simulink model "Phase1_Mark2"  (R2024b)
settings: Solver=ode23tb  StartTime=0.0  StopTime=inf  FixedStep=.001  RelTol=1e-1
model workspace (MAT data in the model file):
  A_mu = 10
  B_reff = 8.386
  CONVERTER_DATA = [0 0.1 0.2 0.3 0.4 0.5 0.6 0.7 0.8 0.81 0.82 0.83 ... (63 elements, 21x3)]
  Cps = 2
  Cz = 7766.25
  DOWN_TABLE = [0 0 0 0 0 0 5 5 7.5 7.5 15 15 ... (30 elements, 6x5)]
  DOWN_TH_BP = [0 5 40 50 90 100]
  D_reff = 0.25826
  EMAP = [-40 215 245 264 264 267 267 267 267 267 -44 117 ... (110 elements, 10x11)]
  F0z = [6086.4 4324.8]
  F_reff = 0.07394
  F_zmax = 10000
  F_zmin = 100
  F_zo = 4000
  Kz = 48000
  MF : object (value not decoded)
  NCyl = 6
  NE_VEC = [800 1200 1600 2000 2400 2800 3200 3600 4000 4400 4800]
  Pstd = 101325
  Rair = 287
  SUS : object (value not decoded)
  TH_VEC = [0; 20; 30; 40; 50; 60; 70; 80; 90; 100]
  TWAITdn = 1.25
  TWAITup = 0.1
  Tin = [1 2 3 4 5 6 7 8 9 10 2 2 ... (20 elements, 10x2)]
  Tstd = 293.15
  UP_TABLE = [7.5 7.5 15 25 40 40 25 25 35 45 70 80 ... (30 elements, 6x5)]
  UP_TH_BP = [0 25 35 50 90 100]
  VEH : object (value not decoded)
  V_o = 16.7
  V_xlow = 1
  Vd = 0.00346
  WH : object (value not decoded)
  a = 1.515
  alpha_max = 1.5
  alpha_min = -1.5
  b = 1.504
  c_zo = 209651
  epsilon = 0.1
  f_air = [0 0 0 0 0 0 0 0 0 0 0 0 ... (256 elements, 16x16)]
  f_co = [0 0 0 0 0 0 0 0 0 0 0 0 ... (256 elements, 16x16)]
  f_co2 = [0 0 0 0 0 0 0 0 0 0 0 0 ... (256 elements, 16x16)]
  f_eff = [352.135682859 352.135682859 320.724378192 303.655312657 295.930136708 291.240087194 291.240271258 291.240312459 291.240275452 291.240198499 291.240100781 291.240018769 ... (256 elements, 16x16)]
  f_fuel = [0 0 0 0 0 0 0 0 0 0 0 0 ... (256 elements, 16x16)]
  f_hc = [0 0 0 0 0 0 0 0 0 0 0 0 ... (256 elements, 16x16)]
  f_nox = [0 0 0 0 0 0 0 0 0 0 0 0 ... (256 elements, 16x16)]
  f_pm = [0 0 0 0 0 0 0 0 0 0 0 0 ... (256 elements, 16x16)]
  f_susp_axl_bp = [1 2]
  f_susp_dz_bp = [-4 -0.14 -0.13 -0.12 -0.11 -0.1 -0.09 -0.08 -0.07 -0.06 -0.05 -0.04 ... (31 elements, 1x31)]
  f_susp_dzdot_bp = [-4 -0.14 -0.13 -0.12 -0.11 -0.1 -0.09 -0.08 -0.07 -0.06 -0.05 -0.04 ... (31 elements, 1x31)]
  f_susp_fmz = [-213379.591456 -28099.591456 -27619.591456 -27139.591456 -26659.591456 -26179.591456 -25699.591456 -25219.591456 -24739.591456 -24259.591456 -23779.591456 -23299.591456 ... (468968 elements, 31x31x61x2x4)]
  f_susp_geom = [-0.832564012244 0.043269987756 0.045538987756 0.047807987756 0.050076987756 0.052345987756 0.054614987756 0.056883987756 0.059152987756 0.061421987756 0.063690987756 0.065959987756 ... (11346 elements, 31x61x2x3)]
  f_susp_strgdelta_bp = [-0.523598775598 -0.506145483078 -0.488692190558 -0.471238898038 -0.453785605519 -0.436332312999 -0.418879020479 -0.401425727959 -0.383972435439 -0.366519142919 -0.349065850399 -0.331612557879 ... (61 elements, 1x61)]
  f_tbrake = [0 76.8593923996 105.140482948 131.533638111 157.926793274 176.658631717 176.65727296 176.656856686 176.656879077 176.657093756 176.657404516 176.65772406 ... (256 elements, 16x16)]
  f_tbrake_n_bpt = [0 649.519052838 912.419621844 1175.32019085 1438.22075986 1701.12132886 1964.02189787 2226.92246687 2489.82303588 2752.72360489 3015.62417389 3278.5247429 ... (16 elements, 1x16)]
  f_tbrake_t_bpt = [0 34.6410161514 61.0341713143 87.4273264773 113.82048164 140.213636803 166.606791966 192.999947129 219.393102292 245.786257455 272.179412618 298.572567781 ... (16 elements, 1x16)]
  f_texh = [766.752464599 766.752464599 786.17542386 801.679939032 884.591982581 910.574397722 910.571871054 910.570774534 910.570601632 910.570821151 910.571247242 910.571639815 ... (256 elements, 16x16)]
  f_twc_eff_co = [0.17 0.25 0.45 0.99 0.99 0.99 0.99]
  f_twc_eff_hc = [0.21 0.375 0.75 0.98 0.98 0.98 0.98]
  f_twc_eff_lam = [0.909090909 0.944055944 0.979020979 1 1.013986014 1.048951049 1.083916084]
  f_twc_eff_nox = [0.98 0.98 0.98 0.97 0.05 0.02 0]
  h = 0.134
  k_z = 50
  kappa_max = 1.5
  kappa_min = -1.5
  lam_Cx = 1
  lam_Cy = 1
  lam_Cz = 1
  lam_Ex = 1
  lam_Ey = 1
  lam_F_zo = 1
  lam_Hx = 1
  lam_Hy = 1
  lam_Kxkappa = 1
  lam_Kyalpha = 1
  lam_Kygamma = 1
  lam_Kzgamma = 1
  lam_Mr = 1
  lam_Mx = 1
  lam_My = 1
  lam_S = 1
  lam_VMx = 1
  lam_Vx = 1
  lam_Vy = 1
  lam_Vykappa = 1
  lam_muV = 0
  lam_mux = 1
  lam_muy = 1
  lam_t = 1
  lam_xalpha = 1
  lam_ykappa = 1
  numWheel = 4
  p_Cx1 = 1.579
  p_Cy1 = 1.3332
  p_Dx1 = 1.0422
  p_Dx2 = -0.08285
  p_Dx3 = 0
  p_Dy1 = 0.8784
  p_Dy2 = -0.06445
  p_Dy3 = 0
  p_Ex1 = 0.11185
  p_Ex2 = 0.3127
  p_Ex3 = 0
  p_Ex4 = 0.001603
  p_Ey1 = -0.8227
  p_Ey2 = -0.6062
  p_Ey3 = 0.09825
  p_Ey4 = -6.546
  p_Ey5 = 0
  p_Fz1 = 0.7098
  p_Hx1 = 0.00021585
  p_Hx2 = 0.0011538
  p_Hy1 = -0.0018043
  p_Hy2 = 0.003518
  p_Kx1 = 21.69
  p_Kx2 = 13.774
  p_Kx3 = -0.4119
  p_Ky1 = -15.314
  p_Ky2 = 1.7044
  p_Ky3 = 0.36986
  p_Ky4 = 1.9896
  p_Ky5 = 0
  p_Ky6 = -0.9004
  p_Ky7 = -0.2328
  p_Vx1 = 1.5973e-05
  p_Vx2 = 0.0001043
  p_Vy1 = -0.006642
  p_Vy2 = 0.03597
  p_Vy3 = -0.1621
  p_Vy4 = -0.4908
  p_pmx1 = 0
  p_px1 = -0.3489
  p_px2 = 0.382
  p_px3 = -0.09634
  p_px4 = 0.06447
  p_py1 = -0.6249
  p_py2 = -0.06535
  p_py3 = -0.1668
  p_py4 = 0.2834
  p_py5 = 0
  path : object (value not decoded)
  pio = 220000
  q_Fcx = 0
  q_Fz2 = 15.4
  q_Fzy = 0
  q_reo = 0.9974
  q_sx1 = -0.007764
  q_sx10 = 0.2824
  q_sx11 = 5.349
  q_sx12 = 0
  q_sx13 = 0
  q_sx14 = 0
  q_sx2 = 1.1915
  q_sx3 = 0.013948
  q_sx4 = 4.912
  q_sx5 = 1.02
  q_sx6 = 22.83
  q_sx7 = 0.7104
  q_sx8 = -0.023393
  q_sx9 = 0.6581
  q_sy1 = 0.00702
  q_sy2 = 0
  q_sy3 = 0.001515
  q_sy4 = 8.514e-05
  q_sy5 = 0
  q_sy6 = 0
  q_sy7 = 0.9008
  q_sy8 = -0.4089
  q_v1 = 0.0007742
  q_v2 = 0.04667
  r_Bx1 = 12.531
  r_Bx2 = 9.532
  r_Bx3 = 0
  r_By1 = 10.615
  r_By2 = 7.705
  r_By3 = 3.433e-06
  r_By4 = 0
  r_Cx1 = 1.019
  r_Cy1 = 1.0585
  r_Ex1 = -0.4487
  r_Ex2 = -0.4726
  r_Ey1 = 0.3132
  r_Ey2 = 7.63e-06
  r_Hx1 = 0.0002374
  r_Hy1 = 0.011646
  r_Hy2 = 7.63e-06
  r_Vy1 = 0.05654
  r_Vy2 = 7.63e-06
  r_Vy3 = 0
  r_Vy4 = 99.9
  r_Vy5 = 2
  r_Vy6 = 15.814
  r_o = 0.3135
  reqTmaxT = [nan 0.285774810084 0.647179872268 nan nan nan nan nan nan nan nan nan ... (168 elements, 21x8)]
  vehSpd = [0 2.77777777778 5.55555555556 8.33333333333 11.1111111111 13.8888888889 16.6666666667 19.4444444444 22.2222222222 25 27.7777777778 30.5555555556 ... (21 elements, 1x21)]
  vehWidth = 2
  w = 1
symbols that are objects in the model workspace (value not decoded): VEH
undefined symbols (not defined in the file or in its folder): Fzz, Fzzdot, InertFrm, pFz, psi, vdyntiremask, x_o, zdotFz, zFz
(part 13 of 24)

== system Phase1_Mark2/Vehicle Body 3DOF External Longitudinal Wheels/Dual/Vehicle Body 3DOF Dual Track/Signal Routing/Signal Routing Dual/state2bus ==
  x : Inport
  y : Inport  Port=2
  Xo : Inport  Port=3
  Angle Wrap : Subsystem  Variant=on  VariantControlMode=label  VariantControl=Variant1  LabelModeActiveChoice=Wrap
  Body Slip : Subsystem
  Bus Creator1 : BusCreator  Inputs=6
  Bus Creator{3,6..7,10..11,13..14} (7 alike) : BusCreator  Inputs=3
  Bus Creator15 : BusCreator  Inputs=6
  Bus Creator2 : BusCreator  Inputs=1
  COMB2I : MATLAB Function  TreatAsAtomicUnit=on
  Constant{,1..10} (11 alike) : Constant  Value=0
  Demux{1..2,4,6} (4 alike) : Demux  Outputs=2
  Demux3 : Demux  Outputs=3
  Demux5 : Demux  Outputs=3
  Integrator : Integrator  InitialConditionSource=external
  Rotation Angles to Direction Cosine Matrix : Subsystem  mask(Ang2DCM){rotationOrder=ZYX, aMode=aMode}
      mask prompts: rotationOrder "shared_aeroblks:sharedaeroblktransform:blockAng2DCMParamRotationOrder"
      mask help: shared_aeroblks:sharedaeroblktransform:blockAng2DCMDesc
      mask init:
      | if aerosharedtest(gcb)
      |     ports=aerosharedicon('sharedang2dcm');
      | else
      |     ports=sharedautoicon('sharedang2dcm');
      | end
      settings: AttributesFormatString=Rotation Order: %<rotationOrder>
      mask Help: eval('if license(''test'',''Aerospace_Blockset'')aerosharedhelp(''rotation_angles_to_direction_cosine_matrix'');elseif license(''test'',''Powertrain_Blockset'')sharedautohelp(''rotation_angles_to_direction_cosine_matrix'');end')
      mask TypeOptions rotationOrder: shared_aeroblks:sharedaeroblktransform:blockParamComboZYX | shared_aeroblks:sharedaeroblktransform:blockParamComboZYZ | shared_aeroblks:sharedaeroblktransform:blockParamComboZXY | shared_aeroblks:sharedaeroblktransform:blockParamComboZXZ | shared_aeroblks:sharedaeroblktransform:blockParamComboYXZ | shared_aeroblks:sharedaeroblktransform:blockParamComboYXY | shared_aeroblks:sharedaeroblktransform:blockParamComboYZX | shared_aeroblks:sharedaeroblktransform:blockParamComboYZY | shared_aeroblks:sharedaeroblktransform:blockParamComboXYZ | shared_aeroblks:sharedaeroblktransform:blockParamComboXYX | shared_aeroblks:sharedaeroblktransform:blockParamComboXZY | shared_aeroblks:sharedaeroblktransform:blockParamComboXZX
      mask DialogControl rotationOrder Prompt: Rotation order:
      mask Display:
      | port_label('input',1,'[R_1,R_2,R_3]','texmode','on')
      | port_label('output',1,'DCM_{be}','texmode','on')
  Selector : Selector  InputPortWidth=3  IndexOptions=Index vector (dialog)  Indices=[3 2 1]  OutputSizes=1
  Selector1 : Selector  IndexOptions=Index vector (dialog)  Indices=[3]  OutputSizes=1
  Selector2 : Selector  IndexOptions=Index vector (dialog)  Indices=[3,1,2]  OutputSizes=1
  Selector4 : Selector  IndexOptions=Index vector (dialog)  Indices=[4,1,2]  OutputSizes=1
  Selector5 : Selector  IndexOptions=Index vector (dialog)  Indices=[1,2]  OutputSizes=1
  Signal Specification : SignalSpecification  Unit=gn
  Signal Specification1 : SignalSpecification  Unit=rad/s
  Signal Specification{4..6,10..12} (6 alike) : SignalSpecification  Unit=m/s
  Signal Specification13 : SignalSpecification  Unit=m
  Signal Specification14 : SignalSpecification  Unit=m
  Signal Specification15 : SignalSpecification  Unit=m
  Signal Specification16 : SignalSpecification  Unit=m/s^2
  Signal Specification17 : SignalSpecification  Unit=m/s^2
  Signal Specification18 : SignalSpecification  Unit=m/s^2
  Signal Specification19 : SignalSpecification  Unit=rad/s^2
  Signal Specification2 : SignalSpecification  Unit=rad/s
  Signal Specification20 : SignalSpecification  Unit=rad/s^2
  Signal Specification21 : SignalSpecification  Unit=rad/s^2
  Signal Specification3 : SignalSpecification  Unit=rad/s
  Signal Specification7 : SignalSpecification  Unit=rad
  Signal Specification8 : SignalSpecification  Unit=rad
  Signal Specification9 : SignalSpecification  Unit=rad
  xddot2ax : Subsystem
  COM_I : Outport  VectorParamsAs1DForOutWhenUnconnected=off
  COM_B : Outport  Port=2  VectorParamsAs1DForOutWhenUnconnected=off
  wires:
  Rotation Angles to Direction Cosine Matrix/1(Out1) -> Bus Creator15/6  "DCM"
  Selector/1 -> Rotation Angles to Direction Cosine Matrix/1(In1)
  [angles] -> Selector/1
  Angle Wrap/1(" y") -> Signal Specification7/1
  Constant10/1 -> Signal Specification20/1
  Bus Creator3/1 -> Bus Creator15/5  "AngAcc"
  Constant9/1 -> Signal Specification19/1
  Signal Specification20/1 -> Bus Creator3/1  "pdot"
  Selector1/1 -> Signal Specification21/1
  Signal Specification19/1 -> Bus Creator3/2  "qdot"
  Signal Specification21/1 -> Bus Creator3/3  "rdot"
  Xo/1 -> Integrator/2
  Bus Creator2/1 -> Bus Creator15/2  "Ang"
  Body Slip/1(Beta) -> Bus Creator2/1  "Beta"
  Demux6/2 -> Signal Specification17/1
  Demux6/1 -> Signal Specification16/1
  Signal Specification16/1 -> Bus Creator1/4  "xddot"
  Signal Specification18/1 -> Bus Creator1/6  "zddot"
  Signal Specification17/1 -> Bus Creator1/5  "yddot"
  Bus Creator1/1 -> Bus Creator15/4  "Acc"
  xddot2ax/1(ax) -> Bus Creator1/1  "ax"
  Demux5/1 -> xddot2ax/1(r), Signal Specification1/1  "r"
  xddot2ax/2(ay) -> Bus Creator1/2  "ay"
  Selector5/1 -> Demux6/1, Demux4/1
  Demux4/2 -> xddot2ax/5(yddot)  "yddot"
  Constant3/1 -> Signal Specification18/1  "zddot"
  Signal Specification/1 -> Bus Creator1/3  "az"
  Demux5/3 -> xddot2ax/3(ydot)  "ydot"
  Constant1/1 -> Signal Specification/1  "az"
  Selector4/1 -> Demux5/1
  Demux4/1 -> xddot2ax/4(xddot)  "xddot"
  Demux5/2 -> xddot2ax/2(xdot)  "xdot"
  y/1 -> Selector5/1, Selector1/1
  Demux2/1 -> Signal Specification14/1
  Demux2/2 -> Signal Specification15/1
  Constant/1 -> Signal Specification13/1
  Demux1/1 -> Signal Specification11/1
  Demux1/2 -> Signal Specification12/1
  Constant8/1 -> Signal Specification10/1
  Constant2/1 -> Signal Specification9/1
  Constant7/1 -> Signal Specification8/1
  Demux3/1 -> Angle Wrap/1("u ")
  Demux3/3 -> Signal Specification6/1
  Demux3/2 -> Signal Specification5/1
  Constant6/1 -> Signal Specification4/1
  Constant4/1 -> Signal Specification3/1
  Constant5/1 -> Signal Specification2/1
  Signal Specification1/1 -> Bus Creator13/3  "r"
  x/1 -> Selector4/1, Body Slip/1(x), Selector2/1, COMB2I/1(x)
  Signal Specification10/1 -> Bus Creator6/3  "Zdot"
  Signal Specification4/1 -> Bus Creator14/3  "zdot"
  Signal Specification11/1 -> Bus Creator6/1  "Xdot"
  Signal Specification15/1 -> Bus Creator10/2  "Y"
  Bus Creator13/1 -> Bus Creator15/3  "AngVel"
  Signal Specification13/1 -> Bus Creator10/3  "Z"
  Signal Specification14/1 -> Bus Creator10/1  "X"
  Signal Specification9/1 -> Bus Creator11/1  "phi"
  Bus Creator7/1 -> COM_I/1  "COM_I"
  Signal Specification3/1 -> Bus Creator13/1  "p"
  Bus Creator14/1 -> Bus Creator15/1  "Vel"
  Bus Creator6/1 -> Bus Creator7/2  "Vel"
  Bus Creator10/1 -> Bus Creator7/1  "Disp"
  Signal Specification8/1 -> Bus Creator11/2  "theta"
  Selector2/1 -> Demux3/1
  Signal Specification12/1 -> Bus Creator6/2  "Ydot"
  Signal Specification2/1 -> Bus Creator13/2  "q"
  Bus Creator15/1 -> COM_B/1  "COM_B"
  Signal Specification5/1 -> Bus Creator14/1  "xdot"
  Bus Creator11/1 -> Bus Creator7/3, [angles]  "Ang"
  Signal Specification6/1 -> Bus Creator14/2  "ydot"
  Integrator/1 -> Demux2/1
  COMB2I/1(y) -> Integrator/1, Demux1/1
  Signal Specification7/1 -> Bus Creator11/3  "psi"

== system Phase1_Mark2/Vehicle Body 3DOF External Longitudinal Wheels/Dual/Vehicle Body 3DOF Dual Track/sigma/sigma/relaxation front ==
  alpha : Inport
  V : Inport  Port=2
  sigma : Inport  Port=3
  Product1 : Product  Inputs=**/  InputSameDT=on  RndMeth=Zero  SaturateOnIntegerOverflow=on  OutDataTypeStr=Inherit: Same as first input
  Sum : Sum  Inputs=-+|  InputSameDT=on  SaturateOnIntegerOverflow=on  OutDataTypeStr=Inherit: Same as first input
  lateral : Integrator
  alpha_sig : Outport  VectorParamsAs1DForOutWhenUnconnected=off
  wires:
  lateral/1 -> alpha_sig/1, Sum/1
  sigma/1 -> Product1/3
  Sum/1 -> Product1/1
  Product1/1 -> lateral/1
  V/1 -> Product1/2
  alpha/1 -> Sum/2

== system Phase1_Mark2/Vehicle Body 3DOF External Longitudinal Wheels/Dual/Vehicle Body 3DOF Dual Track/sigma/sigma/relaxation rear ==
  alpha : Inport
  V : Inport  Port=2
  sigma : Inport  Port=3
  Product1 : Product  Inputs=**/  InputSameDT=on  RndMeth=Zero  SaturateOnIntegerOverflow=on  OutDataTypeStr=Inherit: Same as first input
  Sum : Sum  Inputs=-+|  InputSameDT=on  SaturateOnIntegerOverflow=on  OutDataTypeStr=Inherit: Same as first input
  lateral : Integrator
  alpha_sig : Outport  VectorParamsAs1DForOutWhenUnconnected=off
  wires:
  alpha/1 -> Sum/2
  V/1 -> Product1/2
  Product1/1 -> lateral/1
  Sum/1 -> Product1/1
  sigma/1 -> Product1/3
  lateral/1 -> alpha_sig/1, Sum/1

== system Phase1_Mark2/Vehicle Body 3DOF External Longitudinal Wheels/Dual/Vehicle Body 3DOF Dual Track/sigma/sigma dual/relaxation ==
  alpha : Inport
  V : Inport  Port=2
  sigma : Inport  Port=3
  Product1 : Product  Inputs=**/  InputSameDT=on  RndMeth=Zero  SaturateOnIntegerOverflow=on  OutDataTypeStr=Inherit: Same as first input
  Sum : Sum  Inputs=-+|  InputSameDT=on  SaturateOnIntegerOverflow=on  OutDataTypeStr=Inherit: Same as first input
  lateral : Integrator
  alpha_sig : Outport  VectorParamsAs1DForOutWhenUnconnected=off
  wires:
  alpha/1 -> Sum/2
  V/1 -> Product1/2
  Product1/1 -> lateral/1
  Sum/1 -> Product1/1
  sigma/1 -> Product1/3
  lateral/1 -> Sum/1, alpha_sig/1

== system Phase1_Mark2/Longitudinal Wheels 4DOF/Tires/Fiala/Fiala Tire/Fiala/Rolling/ISO ==
  "Omega " : Inport
  Fz : Inport  Port=2
  Re : Inport  Port=3
  Tamb : Inport  Port=4
  MATLAB Function : MATLAB Function  TreatAsAtomicUnit=on
  My : Outport  VectorParamsAs1DForOutWhenUnconnected=off
  wires:
  Fz/1 -> MATLAB Function/1(Fz)
  "Omega "/1 -> MATLAB Function/2(omega)
  Tamb/1 -> MATLAB Function/3(Tamb)
  Re/1 -> MATLAB Function/4(Re)
  MATLAB Function/1(My) -> My/1

== system Phase1_Mark2/Longitudinal Wheels 4DOF/Tires/Fiala/Fiala Tire/Fiala/Rolling/MagicFormula ==
  "Omega " : Inport
  Fz : Inport  Port=2
  Vx : Inport  Port=3
  Fx : Inport  Port=4
  gamma : Inport  Port=5
  Prs : Inport  Port=6
  MATLAB Function : MATLAB Function  TreatAsAtomicUnit=on
  My : Outport  VectorParamsAs1DForOutWhenUnconnected=off
  wires:
  "Omega "/1 -> MATLAB Function/1(Omega)
  Fz/1 -> MATLAB Function/3(Fz)
  Fx/1 -> MATLAB Function/2(Fx)
  Vx/1 -> MATLAB Function/4(Vx)
  Prs/1 -> MATLAB Function/5(press)
  gamma/1 -> MATLAB Function/6(gamma)
  MATLAB Function/1(My) -> My/1

== system Phase1_Mark2/Longitudinal Wheels 4DOF/Tires/Fiala/Fiala Tire/Fiala/Rolling/Mapped ==
  "Omega " : Inport
  Fz : Inport  Port=2
  Vx : Inport  Port=3
  MATLAB Function : MATLAB Function  TreatAsAtomicUnit=on
  My : Outport  VectorParamsAs1DForOutWhenUnconnected=off
  wires:
  "Omega "/1 -> MATLAB Function/1(omega)
  Fz/1 -> MATLAB Function/2(Fz)
  Vx/1 -> MATLAB Function/3(Vx)
  MATLAB Function/1(My) -> My/1

== system Phase1_Mark2/Longitudinal Wheels 4DOF/Tires/Fiala/Fiala Tire/Fiala/Rolling/None ==
  "Omega " : Inport
  Gain : Gain  Gain=0
  My : Outport  VectorParamsAs1DForOutWhenUnconnected=off
  wires:
  Gain/1 -> My/1
  "Omega "/1 -> Gain/1

== system Phase1_Mark2/Longitudinal Wheels 4DOF/Tires/Fiala/Fiala Tire/Fiala/Rolling/Simple ==
  "Omega " : Inport
  Fz : Inport  Port=2
  Re : Inport  Port=3
  Prs : Inport  Port=4
  Vx : Inport  Port=5
  Abs : Abs  ZeroCross=off  SaturateOnIntegerOverflow=off
  Add : Sum  Inputs=+++
  Constant1 : Constant  Value=PRESMIN
  Constant2 : Constant  Value=aMy
  Constant3 : Constant  Value=FZMIN
  Constant4 : Constant  Value=betaMy
  Constant5 : Constant  Value=alphaMy
  Gain1 : Gain  Gain=4
  Gain2 : Gain  Gain=bMy
  Gain3 : Gain  Gain=cMy
  Max : MinMax  Function=max  Inputs=2
  Max1 : MinMax  Function=max  Inputs=2
  Power : Math  Operator=pow  SignedPower=on
  Power1 : Math  Operator=pow  SignedPower=on
  Product : Product  Inputs=5
  Product1 : Product
  Trigonometric Function : Trigonometry  Operator=tanh
  Unary Minus : UnaryMinus
  My : Outport  VectorParamsAs1DForOutWhenUnconnected=off
  wires:
  Constant3/1 -> Max1/2
  Max1/1 -> Power/1
  Constant1/1 -> Max/2
  Max/1 -> Power1/1
  Fz/1 -> Max1/1
  Gain1/1 -> Trigonometric Function/1
  Product/1 -> Unary Minus/1
  Trigonometric Function/1 -> Product/2
  "Omega "/1 -> Gain1/1
  Unary Minus/1 -> My/1
  Abs/1 -> Gain2/1
  Product1/1 -> Gain3/1
  Constant2/1 -> Add/1
  Gain2/1 -> Add/2
  Gain3/1 -> Add/3
  Re/1 -> Product/3
  Add/1 -> Product/1
  Prs/1 -> Max/1
  Constant4/1 -> Power/2
  Constant5/1 -> Power1/2
  Power/1 -> Product/4
  Power1/1 -> Product/5
  Vx/1 -> Product1/2, Product1/1, Abs/1

== system Phase1_Mark2/Longitudinal Wheels 4DOF/Tires/Fiala/Fiala Tire/Vertical DOF/Mapped Vertical DOF/Vertical Wheel and Unsprung Mass Mapped Response ==
  GroundInput : Inport
  SuspensionForces : Inport  Port=2
  TirePrs : Inport  Port=3
  Damping : Lookup_n-D  BreakpointsForDimension1=pFz  BreakpointsForDimension2=zdotFz  Table=Fzzdot  InternalRulePriority=Speed  RndMeth=Simplest
      settings: InputPortMap=u0,u1
  Fg : Constant  Value=g.*m
  Gain1 : Gain  Gain=1./m  SaturateOnIntegerOverflow=on  OutDataTypeStr=Inherit: Same as input  ParamDataTypeStr=Inherit: Same as input
  "Integrator, Second-Order" : SecondOrderIntegrator  ICX=-zo  ICDXDT=-zdoto
  Saturation : Saturate  UpperLimit=inf  LowerLimit=0
  Stiffness : Lookup_n-D  BreakpointsForDimension1=pFz  BreakpointsForDimension2=zFz  Table=Fzz  InternalRulePriority=Speed  RndMeth=Simplest
      settings: InputPortMap=u0,u1
  Sum1 : Sum  InputSameDT=on  SaturateOnIntegerOverflow=on  OutDataTypeStr=Inherit: Same as first input
  Sum2 : Sum  Inputs=--+  InputSameDT=on  SaturateOnIntegerOverflow=on  OutDataTypeStr=Inherit: Same as first input
  Sum6 : Sum  Inputs=+-  InputSameDT=on  SaturateOnIntegerOverflow=on  OutDataTypeStr=Inherit: Same as first input
  Unary Minus : UnaryMinus
  Unary Minus1 : UnaryMinus
  Unary Minus2 : UnaryMinus
  rhoz : Outport  VectorParamsAs1DForOutWhenUnconnected=off
  z : Outport  Port=2  VectorParamsAs1DForOutWhenUnconnected=off
  zdot : Outport  Port=3  VectorParamsAs1DForOutWhenUnconnected=off
  FzTire : Outport  Port=4  VectorParamsAs1DForOutWhenUnconnected=off
  zddot : Outport  Port=5  VectorParamsAs1DForOutWhenUnconnected=off
  FzDamp : Outport  Port=6  VectorParamsAs1DForOutWhenUnconnected=off
  FzStiff : Outport  Port=7  VectorParamsAs1DForOutWhenUnconnected=off
  wires:
  [FzStiff] -> FzStiff/1
  Gain1/1 -> "Integrator, Second-Order"/1, zddot/1
  TirePrs/1 -> Stiffness/1, Damping/1
  Unary Minus1/1 -> zdot/1
  "Integrator, Second-Order"/2 -> Unary Minus1/1, Damping/2
  Unary Minus2/1 -> z/1
  Unary Minus/1 -> rhoz/1
  Damping/1 -> FzDamp/1, Sum1/2
  Sum1/1 -> Sum2/3, FzTire/1
  Stiffness/1 -> Sum1/1, [FzStiff]
  Fg/1 -> Sum2/1
  Saturation/1 -> Unary Minus/1, Stiffness/2
  GroundInput/1 -> Sum6/1
  "Integrator, Second-Order"/1 -> Sum6/2, Unary Minus2/1  "Zw"
  Sum2/1 -> Gain1/1
  SuspensionForces/1 -> Sum2/2
  Sum6/1 -> Saturation/1

== system Phase1_Mark2/Longitudinal Wheels 4DOF/Tires/Fiala/Fiala Tire/Wheel Module/Brakes/Disk Brake ==
  BrkPrs : Inport
  Omega : Inport  Port=2
  Disk Brake : Subsystem  mask{disk_abore=disk_abore, num_pads=num_pads, Rm=Rm, mu_kinetic=mu_kinetic}
      mask prompts: disk_abore "Disk brake actuator bore, disk_abore [m]:"; num_pads "Number of pads, num_pads [-]:"; Rm "Brake pad mean radius, Rm [m]:"; mu_kinetic "Kinetic friction coefficient, mu_kinetic [-]:"
      mask help: Implements a disk brake pressure to torque transformation model based on the number of brake pads, brake actuator bore area, mean pad force application radius, and static friction coefficient.
      mask Help: Provide number of brake pads, pad area, static friction coefficient, and dynamic friction coefficient.
  MyBrk : Outport  VectorParamsAs1DForOutWhenUnconnected=off
  wires:
  BrkPrs/1 -> Disk Brake/1(Brake Pressure)
  Omega/1 -> Disk Brake/2(Wheel angular velocity)
  Disk Brake/1(Brake Torque) -> MyBrk/1

== system Phase1_Mark2/Longitudinal Wheels 4DOF/Tires/Fiala/Fiala Tire/Wheel Module/Brakes/Drum Brake ==
  BrkPrs : Inport
  Omega : Inport  Port=2
  Drum Brake : Subsystem  mask{drum_abore=drum_abore, mu_kinetic=mu_kinetic, drum_a=drum_a, drum_c=drum_c, drum_r=drum_r, drum_theta1=drum_theta1, drum_theta2=drum_theta2}
      mask prompts: drum_abore "Drum brake actuator bore, drum_abore [m]:"; mu_kinetic "Kinetic friction coefficient, mu_kinetic [-]:"; drum_a "Shoe pin to drum center distance, drum_a [m]:"; drum_c "Shoe pin center to force application point distance, drum_c [m]:"; drum_r "Drum internal radius, drum_r [m]:"; drum_theta1 "Shoe pin to pad start angle, drum_theta1 [deg]:"; drum_theta2 "Shoe pin to pad end angle, drum_theta2 [deg]:"
      mask help: Implements a drum brake pressure to torque transformation model based on the drum and shoe geometry parameters provided by the user.
  MyBrk : Outport  VectorParamsAs1DForOutWhenUnconnected=off
  wires:
  Drum Brake/1(Brake Torque) -> MyBrk/1
  Omega/1 -> Drum Brake/2(Wheel angular velocity)
  BrkPrs/1 -> Drum Brake/1(Brake Pressure)

== system Phase1_Mark2/Longitudinal Wheels 4DOF/Tires/Fiala/Fiala Tire/Wheel Module/Brakes/Mapped Brake ==
  BrkPrs : Inport
  Omega : Inport  Port=2
  Cont LPF : Subsystem  mask{wc=200*2*pi, AbsoluteTolerance=auto, aMode=aMode}
      mask prompts: wc "Cutoff frequency, wc [rad/s]"; AbsoluteTolerance "Simulink:blkprm_prompts:ContinuousStateAbsoluteTolerance"
      mask init:
      | [~]=autosharedicon('autolibutils',gcb,0);
      mask TypeOptions AbsoluteTolerance: Integrator1/AbsoluteTolerance
      mask DialogControl AbsoluteTolerance Prompt: Absolute tolerance:
      mask Display: fprintf('LPF')
  Mapped Brake : Subsystem  mask{brake_p_bpt=brake_p_bpt, brake_n_bpt=brake_n_bpt, f_brake_t=f_brake_t}
      mask prompts: brake_p_bpt "Brake actuator pressure breakpoints, brake_p_bpt [bar]:"; brake_n_bpt "Wheel speed breakpoints, brake_n_bpt [rpm]:"; f_brake_t "Brake torque map, f_brake_t [Nm]:"
      mask help: Implements a generic map-based brake pressure to torque transformation model based on brake dynamometer performance data. You can characterize brake torque as a function of brake actuator pressure and wheel speed.
  MyBrk : Outport  VectorParamsAs1DForOutWhenUnconnected=off
  wires:
  Cont LPF/1(y) -> Mapped Brake/2(Wheel angular velocity)
  Omega/1 -> Cont LPF/1(u)
  Mapped Brake/1(Brake Torque) -> MyBrk/1
  BrkPrs/1 -> Mapped Brake/1(Brake Pressure)

== system Phase1_Mark2/Longitudinal Wheels 4DOF/Tires/Fiala/Fiala Tire/Wheel Module/Brakes/No Brake ==
  BrkPrs : Inport
  Omega : Inport  Port=2
  Ground : Ground
  Terminator : Terminator
  Terminator1 : Terminator
  MyBrk : Outport  VectorParamsAs1DForOutWhenUnconnected=off
  wires:
  BrkPrs/1 -> Terminator/1
  Ground/1 -> MyBrk/1
  Omega/1 -> Terminator1/1

== system Phase1_Mark2/Longitudinal Wheels 4DOF/Tires/Fiala/Fiala Tire/Wheel Module/Clutch/Clutch Partitioned Parameters ==
  Tout : Inport  Partition=on  PartitionDimension=1  PartitionWidth=1  PartitionOffset=0
  Tfmaxs : Inport  Port=2  Partition=on  PartitionDimension=1  PartitionWidth=1  PartitionOffset=0
  Tfmaxk : Inport  Port=3  Partition=on  PartitionDimension=1  PartitionWidth=1  PartitionOffset=0
  Clutch : Stateflow chart  TreatAsAtomicUnit=on  mask{OmegaTol=pi/30}
  For Each : ForEach  DisableCoverage=on  IterateSubsysMaskParameter=on,on,off,on
  Terminator : Terminator
  Terminator1 : Terminator
  Omega : Outport  ConcatenationDimension=1  VectorParamsAs1DForOutWhenUnconnected=off
  Omegadot : Outport  Port=2  ConcatenationDimension=1  VectorParamsAs1DForOutWhenUnconnected=off
  Myb : Outport  Port=3  ConcatenationDimension=1  VectorParamsAs1DForOutWhenUnconnected=off
  wires:
  Clutch/5(BrkTrq) -> Terminator1/1
  Clutch/2(Omegadot) -> Omegadot/1
  Clutch/1(Omega) -> Omega/1
  Clutch/3(Myb) -> Myb/1
  Clutch/4(ReactionTorque) -> Terminator/1
  Tfmaxk/1 -> Clutch/3(Tfmaxk)
  Tfmaxs/1 -> Clutch/2(Tfmaxs)
  Tout/1 -> Clutch/1(Tout)

== system Phase1_Mark2/Longitudinal Wheels 4DOF/Tires/Fiala/Fiala Tire/Wheel Module/Clutch/Clutch Scalar Parameters ==
  Tout : Inport  Partition=on  PartitionDimension=1  PartitionWidth=1  PartitionOffset=0
  Tfmaxs : Inport  Port=2  Partition=on  PartitionDimension=1  PartitionWidth=1  PartitionOffset=0
  Tfmaxk : Inport  Port=3  Partition=on  PartitionDimension=1  PartitionWidth=1  PartitionOffset=0
  Clutch : Stateflow chart  TreatAsAtomicUnit=on  mask{OmegaTol=pi/30}
  For Each : ForEach  DisableCoverage=on  IterateSubsysMaskParameter=off,off,off,off
  Terminator : Terminator
  Terminator1 : Terminator
  Omega : Outport  ConcatenationDimension=1  VectorParamsAs1DForOutWhenUnconnected=off
  Omegadot : Outport  Port=2  ConcatenationDimension=1  VectorParamsAs1DForOutWhenUnconnected=off
  Myb : Outport  Port=3  ConcatenationDimension=1  VectorParamsAs1DForOutWhenUnconnected=off
  wires:
  Clutch/5(BrkTrq) -> Terminator1/1
  Tout/1 -> Clutch/1(Tout)
  Tfmaxs/1 -> Clutch/2(Tfmaxs)
  Tfmaxk/1 -> Clutch/3(Tfmaxk)
  Clutch/4(ReactionTorque) -> Terminator/1
  Clutch/3(Myb) -> Myb/1
  Clutch/1(Omega) -> Omega/1
  Clutch/2(Omegadot) -> Omegadot/1

== system Phase1_Mark2/Longitudinal Wheels 4DOF/Tires/MF/Combined Slip Wheel 2DOF/Vertical DOF/Mapped Vertical DOF/Vertical Wheel and Unsprung Mass Mapped Response ==
  GroundInput : Inport
  SuspensionForces : Inport  Port=2
  TirePrs : Inport  Port=3
  Damping : Lookup_n-D  BreakpointsForDimension1=pFz  BreakpointsForDimension2=zdotFz  Table=Fzzdot  InternalRulePriority=Speed  RndMeth=Simplest
      settings: InputPortMap=u0,u1
  Fg : Constant  Value=g.*m
  Gain1 : Gain  Gain=1./m  SaturateOnIntegerOverflow=on  OutDataTypeStr=Inherit: Same as input  ParamDataTypeStr=Inherit: Same as input
  "Integrator, Second-Order" : SecondOrderIntegrator  ICX=-zo  ICDXDT=-zdoto
  Saturation : Saturate  UpperLimit=inf  LowerLimit=0
  Stiffness : Lookup_n-D  BreakpointsForDimension1=pFz  BreakpointsForDimension2=zFz  Table=Fzz  InternalRulePriority=Speed  RndMeth=Simplest
      settings: InputPortMap=u0,u1
  Sum1 : Sum  InputSameDT=on  SaturateOnIntegerOverflow=on  OutDataTypeStr=Inherit: Same as first input
  Sum2 : Sum  Inputs=--+  InputSameDT=on  SaturateOnIntegerOverflow=on  OutDataTypeStr=Inherit: Same as first input
  Sum6 : Sum  Inputs=+-  InputSameDT=on  SaturateOnIntegerOverflow=on  OutDataTypeStr=Inherit: Same as first input
  Unary Minus : UnaryMinus
  Unary Minus1 : UnaryMinus
  Unary Minus2 : UnaryMinus
  rhoz : Outport  VectorParamsAs1DForOutWhenUnconnected=off
  z : Outport  Port=2  VectorParamsAs1DForOutWhenUnconnected=off
  zdot : Outport  Port=3  VectorParamsAs1DForOutWhenUnconnected=off
  FzTire : Outport  Port=4  VectorParamsAs1DForOutWhenUnconnected=off
  zddot : Outport  Port=5  VectorParamsAs1DForOutWhenUnconnected=off
  FzDamp : Outport  Port=6  VectorParamsAs1DForOutWhenUnconnected=off
  FzStiff : Outport  Port=7  VectorParamsAs1DForOutWhenUnconnected=off
  wires:
  [FzStiff] -> FzStiff/1
  Gain1/1 -> "Integrator, Second-Order"/1, zddot/1
  TirePrs/1 -> Stiffness/1, Damping/1
  Unary Minus1/1 -> zdot/1
  "Integrator, Second-Order"/2 -> Unary Minus1/1, Damping/2
  Unary Minus2/1 -> z/1
  Unary Minus/1 -> rhoz/1
  Damping/1 -> FzDamp/1, Sum1/2
  Sum1/1 -> Sum2/3, FzTire/1
  Stiffness/1 -> Sum1/1, [FzStiff]
  Fg/1 -> Sum2/1
  Saturation/1 -> Unary Minus/1, Stiffness/2
  GroundInput/1 -> Sum6/1
  "Integrator, Second-Order"/1 -> Sum6/2, Unary Minus2/1  "Zw"
  Sum2/1 -> Gain1/1
  SuspensionForces/1 -> Sum2/2
  Sum6/1 -> Saturation/1

== system Phase1_Mark2/Longitudinal Wheels 4DOF/Tires/MF/Combined Slip Wheel 2DOF/Wheel Module/Brakes/Disk Brake ==
  BrkPrs : Inport
  Omega : Inport  Port=2
  Disk Brake : Subsystem  mask{disk_abore=disk_abore, num_pads=num_pads, Rm=Rm, mu_kinetic=mu_kinetic}
      mask prompts: disk_abore "Disk brake actuator bore, disk_abore [m]:"; num_pads "Number of pads, num_pads [-]:"; Rm "Brake pad mean radius, Rm [m]:"; mu_kinetic "Kinetic friction coefficient, mu_kinetic [-]:"
      mask help: Implements a disk brake pressure to torque transformation model based on the number of brake pads, brake actuator bore area, mean pad force application radius, and static friction coefficient.
      mask Help: Provide number of brake pads, pad area, static friction coefficient, and dynamic friction coefficient.
  MyBrk : Outport  VectorParamsAs1DForOutWhenUnconnected=off
  wires:
  BrkPrs/1 -> Disk Brake/1(Brake Pressure)
  Omega/1 -> Disk Brake/2(Wheel angular velocity)
  Disk Brake/1(Brake Torque) -> MyBrk/1

== system Phase1_Mark2/Longitudinal Wheels 4DOF/Tires/MF/Combined Slip Wheel 2DOF/Wheel Module/Brakes/Drum Brake ==
  BrkPrs : Inport
  Omega : Inport  Port=2
  Drum Brake : Subsystem  mask{drum_abore=drum_abore, mu_kinetic=mu_kinetic, drum_a=drum_a, drum_c=drum_c, drum_r=drum_r, drum_theta1=drum_theta1, drum_theta2=drum_theta2}
      mask prompts: drum_abore "Drum brake actuator bore, drum_abore [m]:"; mu_kinetic "Kinetic friction coefficient, mu_kinetic [-]:"; drum_a "Shoe pin to drum center distance, drum_a [m]:"; drum_c "Shoe pin center to force application point distance, drum_c [m]:"; drum_r "Drum internal radius, drum_r [m]:"; drum_theta1 "Shoe pin to pad start angle, drum_theta1 [deg]:"; drum_theta2 "Shoe pin to pad end angle, drum_theta2 [deg]:"
      mask help: Implements a drum brake pressure to torque transformation model based on the drum and shoe geometry parameters provided by the user.
  MyBrk : Outport  VectorParamsAs1DForOutWhenUnconnected=off
  wires:
  Drum Brake/1(Brake Torque) -> MyBrk/1
  Omega/1 -> Drum Brake/2(Wheel angular velocity)
  BrkPrs/1 -> Drum Brake/1(Brake Pressure)

== system Phase1_Mark2/Longitudinal Wheels 4DOF/Tires/MF/Combined Slip Wheel 2DOF/Wheel Module/Brakes/Mapped Brake ==
  BrkPrs : Inport
  Omega : Inport  Port=2
  Cont LPF : Subsystem  mask{wc=200*2*pi, AbsoluteTolerance=auto, aMode=aMode}
      mask prompts: wc "Cutoff frequency, wc [rad/s]"; AbsoluteTolerance "Simulink:blkprm_prompts:ContinuousStateAbsoluteTolerance"
      mask init:
      | [~]=autosharedicon('autolibutils',gcb,0);
      mask TypeOptions AbsoluteTolerance: Integrator1/AbsoluteTolerance
      mask DialogControl AbsoluteTolerance Prompt: Absolute tolerance:
      mask Display: fprintf('LPF')
  Mapped Brake : Subsystem  mask{brake_p_bpt=brake_p_bpt, brake_n_bpt=brake_n_bpt, f_brake_t=f_brake_t}
      mask prompts: brake_p_bpt "Brake actuator pressure breakpoints, brake_p_bpt [bar]:"; brake_n_bpt "Wheel speed breakpoints, brake_n_bpt [rpm]:"; f_brake_t "Brake torque map, f_brake_t [Nm]:"
      mask help: Implements a generic map-based brake pressure to torque transformation model based on brake dynamometer performance data. You can characterize brake torque as a function of brake actuator pressure and wheel speed.
  MyBrk : Outport  VectorParamsAs1DForOutWhenUnconnected=off
  wires:
  Cont LPF/1(y) -> Mapped Brake/2(Wheel angular velocity)
  Omega/1 -> Cont LPF/1(u)
  Mapped Brake/1(Brake Torque) -> MyBrk/1
  BrkPrs/1 -> Mapped Brake/1(Brake Pressure)

== system Phase1_Mark2/Longitudinal Wheels 4DOF/Tires/MF/Combined Slip Wheel 2DOF/Wheel Module/Brakes/No Brake ==
  BrkPrs : Inport
  Omega : Inport  Port=2
  Ground : Ground
  Terminator : Terminator
  Terminator1 : Terminator
  MyBrk : Outport  VectorParamsAs1DForOutWhenUnconnected=off
  wires:
  BrkPrs/1 -> Terminator/1
  Ground/1 -> MyBrk/1
  Omega/1 -> Terminator1/1

== system Phase1_Mark2/Longitudinal Wheels 4DOF/Tires/MF/Combined Slip Wheel 2DOF/Wheel Module/Clutch/Clutch Partitioned Parameters ==
  Tout : Inport  Partition=on  PartitionDimension=1  PartitionWidth=1  PartitionOffset=0
  Tfmaxs : Inport  Port=2  Partition=on  PartitionDimension=1  PartitionWidth=1  PartitionOffset=0
  Tfmaxk : Inport  Port=3  Partition=on  PartitionDimension=1  PartitionWidth=1  PartitionOffset=0
  Clutch : Stateflow chart  TreatAsAtomicUnit=on  mask{OmegaTol=pi/30}
  For Each : ForEach  DisableCoverage=on  IterateSubsysMaskParameter=on,on,off,on
  Terminator : Terminator
  Terminator1 : Terminator
  Omega : Outport  ConcatenationDimension=1  VectorParamsAs1DForOutWhenUnconnected=off
  Omegadot : Outport  Port=2  ConcatenationDimension=1  VectorParamsAs1DForOutWhenUnconnected=off
  Myb : Outport  Port=3  ConcatenationDimension=1  VectorParamsAs1DForOutWhenUnconnected=off
  wires:
  Clutch/5(BrkTrq) -> Terminator1/1
  Clutch/2(Omegadot) -> Omegadot/1
  Clutch/1(Omega) -> Omega/1
  Clutch/3(Myb) -> Myb/1
  Clutch/4(ReactionTorque) -> Terminator/1
  Tfmaxk/1 -> Clutch/3(Tfmaxk)
  Tfmaxs/1 -> Clutch/2(Tfmaxs)
  Tout/1 -> Clutch/1(Tout)

== system Phase1_Mark2/Longitudinal Wheels 4DOF/Tires/MF/Combined Slip Wheel 2DOF/Wheel Module/Clutch/Clutch Scalar Parameters ==
  Tout : Inport  Partition=on  PartitionDimension=1  PartitionWidth=1  PartitionOffset=0
  Tfmaxs : Inport  Port=2  Partition=on  PartitionDimension=1  PartitionWidth=1  PartitionOffset=0
  Tfmaxk : Inport  Port=3  Partition=on  PartitionDimension=1  PartitionWidth=1  PartitionOffset=0
  Clutch : Stateflow chart  TreatAsAtomicUnit=on  mask{OmegaTol=pi/30}
  For Each : ForEach  DisableCoverage=on  IterateSubsysMaskParameter=off,off,off,off
  Terminator : Terminator
  Terminator1 : Terminator
  Omega : Outport  ConcatenationDimension=1  VectorParamsAs1DForOutWhenUnconnected=off
  Omegadot : Outport  Port=2  ConcatenationDimension=1  VectorParamsAs1DForOutWhenUnconnected=off
  Myb : Outport  Port=3  ConcatenationDimension=1  VectorParamsAs1DForOutWhenUnconnected=off
  wires:
  Clutch/5(BrkTrq) -> Terminator1/1
  Tout/1 -> Clutch/1(Tout)
  Tfmaxs/1 -> Clutch/2(Tfmaxs)
  Tfmaxk/1 -> Clutch/3(Tfmaxk)
  Clutch/4(ReactionTorque) -> Terminator/1
  Clutch/3(Myb) -> Myb/1
  Clutch/1(Omega) -> Omega/1
  Clutch/2(Omegadot) -> Omegadot/1

== system Phase1_Mark2/Vehicle Body 3DOF External Longitudinal Wheels/Bicycle/Vehicle Body 3DOF Single Track/Signal Routing/Signal Routing/Lateral 3DOF/Hard Point Coordinate Transform Front ==
  InertFrmCg : Inport
  BdyFrmCg : Inport  Port=2
  Steer : Inport  Port=3
  Add : Sum
  Add1 : Sum
  Add4 : Sum
  Bus Creator{1..3,6,10} (5 alike) : BusCreator  Inputs=3
  Bus Creator7 : BusCreator  Inputs=2
  Bus Selector1 : BusSelector  OutputSignals=Vel.xdot,Vel.ydot,Vel.zdot  OutputAsBus=on
  Bus Selector4 : BusSelector  OutputSignals=Disp.X,Disp.Y,Disp.Z  OutputAsBus=on
  Bus Selector5 : BusSelector  OutputSignals=AngVel.p,AngVel.q,AngVel.r  OutputAsBus=on
  Bus Selector6 : BusSelector  OutputSignals=Vel.Xdot,Vel.Ydot,Vel.Zdot  OutputAsBus=on
  Bus Selector8 : BusSelector  OutputSignals=Ang.phi,Ang.theta,Ang.psi  OutputAsBus=on
  Bus to Vector{,1..4} (5 alike) : BusToVector
  Demux{1..4} (4 alike) : Demux  Outputs=3
  R_T1 : Constant  Value=R_T1
  R_T2 : Constant  Value=R_T2
  R_T3 : Constant  Value=R_T3
  Rotation Angles to Direction Cosine Matrix : Subsystem  mask(Ang2DCM){rotationOrder=ZYX, aMode=aMode}
      mask prompts: rotationOrder "shared_aeroblks:sharedaeroblktransform:blockAng2DCMParamRotationOrder"
      mask help: shared_aeroblks:sharedaeroblktransform:blockAng2DCMDesc
      mask init:
      | if aerosharedtest(gcb)
      |     ports=aerosharedicon('sharedang2dcm');
      | else
      |     ports=sharedautoicon('sharedang2dcm');
      | end
      settings: AttributesFormatString=Rotation Order: %<rotationOrder>
      mask Help: eval('if license(''test'',''Aerospace_Blockset'')aerosharedhelp(''rotation_angles_to_direction_cosine_matrix'');elseif license(''test'',''Powertrain_Blockset'')sharedautohelp(''rotation_angles_to_direction_cosine_matrix'');end')
      mask TypeOptions rotationOrder: shared_aeroblks:sharedaeroblktransform:blockParamComboZYX | shared_aeroblks:sharedaeroblktransform:blockParamComboZYZ | shared_aeroblks:sharedaeroblktransform:blockParamComboZXY | shared_aeroblks:sharedaeroblktransform:blockParamComboZXZ | shared_aeroblks:sharedaeroblktransform:blockParamComboYXZ | shared_aeroblks:sharedaeroblktransform:blockParamComboYXY | shared_aeroblks:sharedaeroblktransform:blockParamComboYZX | shared_aeroblks:sharedaeroblktransform:blockParamComboYZY | shared_aeroblks:sharedaeroblktransform:blockParamComboXYZ | shared_aeroblks:sharedaeroblktransform:blockParamComboXYX | shared_aeroblks:sharedaeroblktransform:blockParamComboXZY | shared_aeroblks:sharedaeroblktransform:blockParamComboXZX
      mask DialogControl rotationOrder Prompt: Rotation order:
      mask Display:
      | port_label('input',1,'[R_1,R_2,R_3]','texmode','on')
      | port_label('output',1,'DCM_{be}','texmode','on')
  Selector1 : Selector  InputPortWidth=3  IndexOptions=Index vector (dialog)  Indices=[3 2 1]  OutputSizes=1
  Signal Specification : SignalSpecification  Unit=m
  Signal Specification1 : SignalSpecification  Unit=m
  Signal Specification2 : SignalSpecification  Unit=m/s
  Signal Specification3 : SignalSpecification  Unit=m/s
  Transpose1 : Math  Operator=transpose  SignedPower=on
  Vector Concatenate : Concatenate  NumInputs=3
  transform to Inertial axes : Subsystem  mask(Vector Transformation){}
      mask Display: disp('L_EB')
  transform to Inertial axes1 : Subsystem  mask(Vector Transformation){}
      mask Display: disp('L_EB')
  wxR : Subsystem  mask(CrossProduct){aMode=aMode}
      mask help: shared_aeroblks:sharedaeroblkutil:blockCrossProductDesc
      mask init:
      | if aerosharedtest(gcb)
      |     aerosharedicon('shared');
      | else
      |     sharedautoicon('shared');
      | end
      mask Help: eval('if license(''test'',''Aerospace_Blockset'')aerosharedhelp(''threebythree_cross_product'');elseif license(''test'',''Powertrain_Blockset'')sharedautohelp(''threebythree_cross_product'');end')
      mask Display:
      | text(.5,.5,'Cross\nProduct\nC = AxB', ...
      | 	'HorizontalAlignment','Center',...
      | 	'VerticalAlignment','middle')
  Inertial : Outport  VectorParamsAs1DForOutWhenUnconnected=off
  Body : Outport  Port=2  VectorParamsAs1DForOutWhenUnconnected=off
  wires:
  Steer/1 -> Bus Creator3/3  "Steer"
  Signal Specification3/1 -> Demux4/1
  Signal Specification2/1 -> Demux2/1
  Signal Specification1/1 -> Demux3/1
  Signal Specification/1 -> Demux1/1
  Vector Concatenate/1 -> Signal Specification1/1, transform to Inertial axes1/1(x y z), wxR/2(B)
  R_T3/1 -> Vector Concatenate/3
  R_T1/1 -> Vector Concatenate/1
  R_T2/1 -> Vector Concatenate/2
  Bus to Vector3/1 -> Add1/2
  Add1/1 -> Signal Specification3/1
  Bus Selector1/1 -> Bus to Vector3/1
  Bus Creator3/1 -> Body/1
  Demux4/2 -> Bus Creator2/2  "ydot"
  Demux3/2 -> Bus Creator1/2  "y"
  Demux3/3 -> Bus Creator1/3  "z"
  Demux3/1 -> Bus Creator1/1  "x"
  Demux4/3 -> Bus Creator2/3  "zdot"
  Demux4/1 -> Bus Creator2/1  "xdot"
  Bus Creator2/1 -> Bus Creator3/2  "Vel"
  Bus Creator1/1 -> Bus Creator3/1  "Disp"
  Bus Creator7/1 -> Inertial/1
  Demux2/2 -> Bus Creator6/2  "Ydot"
  Demux1/2 -> Bus Creator10/2  "Y"
  Demux1/3 -> Bus Creator10/3  "Z"
  Demux1/1 -> Bus Creator10/1  "X"
  Demux2/3 -> Bus Creator6/3  "Zdot"
  Demux2/1 -> Bus Creator6/1  "Xdot"
  Bus Creator6/1 -> Bus Creator7/2  "Vel"
  Bus Creator10/1 -> Bus Creator7/1  "Disp"
  transform to Inertial axes1/1(Ve) -> Add/2
  Bus to Vector4/1 -> Selector1/1
  Bus Selector8/1 -> Bus to Vector4/1
  Rotation Angles to Direction Cosine Matrix/1(Out1) -> Transpose1/1
  Selector1/1 -> Rotation Angles to Direction Cosine Matrix/1(In1)
  Transpose1/1 -> transform to Inertial axes/2(transform coefficients), transform to Inertial axes1/2(transform coefficients)
  wxR/1(C) -> Add1/1, transform to Inertial axes/1(x y z)
  Bus to Vector1/1 -> Add4/1  "Vo"
  transform to Inertial axes/1(Ve) -> Add4/2
  Bus to Vector/1 -> wxR/1(A)
  Bus Selector5/1 -> Bus to Vector/1
  Bus Selector6/1 -> Bus to Vector1/1
  Add4/1 -> Signal Specification2/1  "V_wb"
  Add/1 -> Signal Specification/1
  Bus Selector4/1 -> Bus to Vector2/1
  Bus to Vector2/1 -> Add/1
  InertFrmCg/1 -> Bus Selector4/1, Bus Selector6/1, Bus Selector8/1
  BdyFrmCg/1 -> Bus Selector5/1, Bus Selector1/1

== system Phase1_Mark2/Vehicle Body 3DOF External Longitudinal Wheels/Bicycle/Vehicle Body 3DOF Single Track/Signal Routing/Signal Routing/Lateral 3DOF/Hard Point Coordinate Transform Geometric ==
  InertFrmCg : Inport
  BdyFrmCg : Inport  Port=2
  Hard Point Coordinate Transform External Displacement Beta : Subsystem  mask(Hard Point Coordinate Transform){xdot_tol=xdot_tol, aMode=aMode}
      mask prompts: xdot_tol "Low speed longitudinal velocity tolerance, xdot_tol [m/s]:"
  Vector Concatenate : Concatenate  NumInputs=3
  latOff : Constant  Value=latOff
  longOff : Constant  Value=longOff
  vertOff : Constant  Value=vertOff
  Inert : Outport  VectorParamsAs1DForOutWhenUnconnected=off
  Body : Outport  Port=2  VectorParamsAs1DForOutWhenUnconnected=off
  wires:
  latOff/1 -> Vector Concatenate/2
  longOff/1 -> Vector Concatenate/1
  vertOff/1 -> Vector Concatenate/3
  Hard Point Coordinate Transform External Displacement Beta/1(Inertial) -> Inert/1
  BdyFrmCg/1 -> Hard Point Coordinate Transform External Displacement Beta/2(BdyFrmCg)
  Vector Concatenate/1 -> Hard Point Coordinate Transform External Displacement Beta/3(R)
  Hard Point Coordinate Transform External Displacement Beta/2(Body) -> Body/1
  InertFrmCg/1 -> Hard Point Coordinate Transform External Displacement Beta/1(InertFrmCg)
